simulink model "scheme_echivalente_ex3"  (R2021b)
settings: Solver=VariableStepAuto  StartTime=0.0  StopTime=10.0  RelTol=1e-3
settings Model: Creator=Rares  LastModifiedBy=Rares

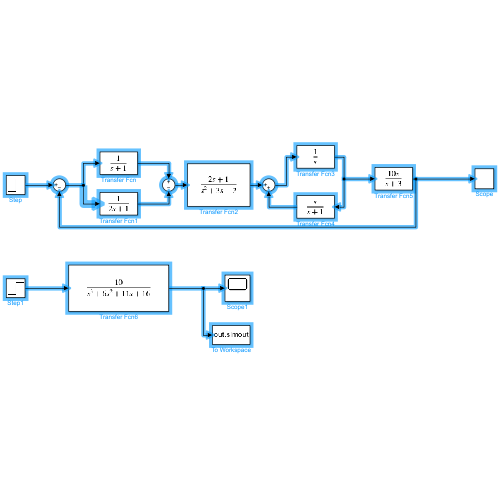
[thumbnail: Simulink's stored preview of the top-level diagram]
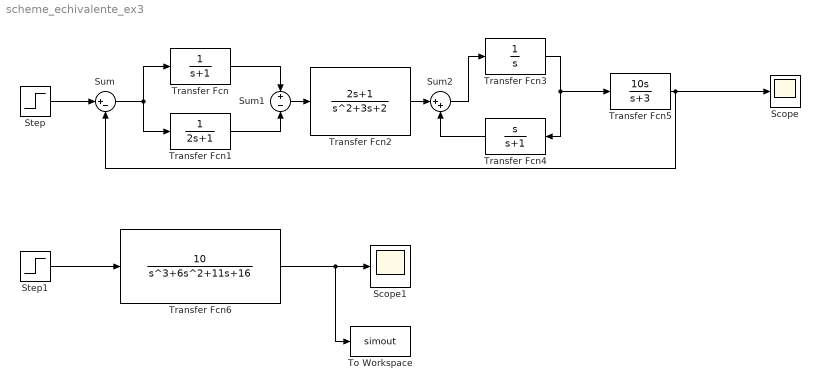
== system scheme_echivalente_ex3 ==
  Scope : Scope
  Scope1 : Scope
  Step : Step  Time=0  SampleTime=0
  Step1 : Step  Time=0  SampleTime=0
  Sum : Sum  Inputs=|+-
  Sum1 : Sum  Inputs=+|-
  Sum2 : Sum  Inputs=|++
  To Workspace : ToWorkspace  VariableName=simout  SaveFormat=Timeseries  SampleTime=-1
  Transfer Fcn : TransferFcn  Denominator=[1 1]
  Transfer Fcn1 : TransferFcn  Denominator=[2 1]
  Transfer Fcn2 : TransferFcn  Numerator=[2 1]  Denominator=[1 3 2]
  Transfer Fcn3 : TransferFcn  Denominator=[1 0]
  Transfer Fcn4 : TransferFcn  Numerator=[1 0]  Denominator=[1 1]
  Transfer Fcn5 : TransferFcn  Numerator=[10 0]  Denominator=[1 3]
  Transfer Fcn6 : TransferFcn  Numerator=[10]  Denominator=[1 6 11 16]
  wires:
  Transfer Fcn5/1 -> Sum/2, Scope/1
  Sum2/1 -> Transfer Fcn3/1
  Transfer Fcn3/1 -> Transfer Fcn5/1, Transfer Fcn4/1
  Step/1 -> Sum/1
  Transfer Fcn4/1 -> Sum2/2
  Step1/1 -> Transfer Fcn6/1
  Transfer Fcn6/1 -> To Workspace/1, Scope1/1
  Sum1/1 -> Transfer Fcn2/1
  Transfer Fcn2/1 -> Sum2/1
  Transfer Fcn/1 -> Sum1/1
  Transfer Fcn1/1 -> Sum1/2
  Sum/1 -> Transfer Fcn1/1, Transfer Fcn/1
